simulink model "main"  (Simulink 8.1)
settings: Solver=ode4  StartTime=0  StopTime=0.2  FixedStep=Ts  MaxStep=1e-6  RelTol=1e-6  AbsTol=1e-6
PreLoadFcn:
  | assignin('base','Ts',[5e-6])
  | Ki=16.61;
  | Kp=0.013;
undefined symbols (not defined in the file): Ts
libraries: simulink x12, powerlib x11
Description:
  | This demonstration illustrates use of the BLDC in a closed-loop
  | speed and voltage control on a 1 kW, 3000 rpm industrial motor
  | 
  | 
  | Copyright 2008-2009 The MathWorks(TM), Inc.
settings Model: Creator=Olivier Tremblay  LastModifiedBy=The  ExtModeAutoUpdateStatusClock=off
settings DataIOCC: SignalLoggingName=sigsOut
settings OptimizationCC: InitFltsAndDblsToZero=on
settings DebuggingCC: SignalResolutionControl=TryResolveAllWithWarning  SolverPrmCheckMsg=none  MultiTaskDSMMsg=warning  MultiTaskCondExecSysMsg=none  UnknownTsInhSupMsg=none  StrictBusMsg=None
settings HardwareCC: TargetUnknown=on
settings RTWCC: IncludeERTFirstTime=on

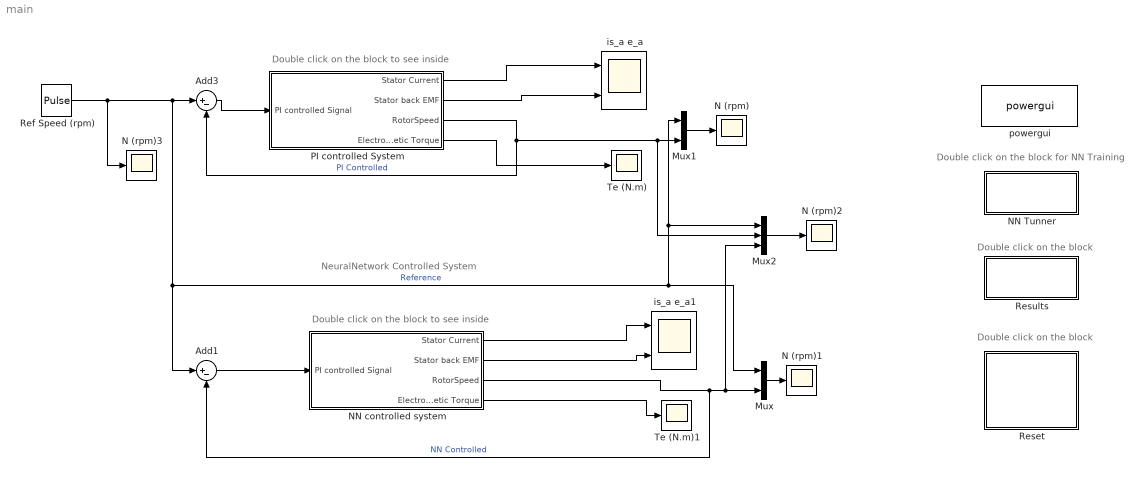
== system main ==
  note: Double click on the block for NN Training
  note: NeuralNetwork Controlled System
  note: Double click on the block to see inside
  note: Double click on the block to see inside
  note: Double click on the block
  note: Double click on the block
  Add1 : Sum  Inputs=|+-
  Add3 : Sum  Inputs=|+-
  Mux : Mux  Inputs=2
  Mux1 : Mux  Inputs=2
  Mux2 : Mux  Inputs=3
  N (rpm){,1..3} (4 alike) : Scope
      N (rpm) settings: TimeRange=0.2  YMin=0  YMax=3500  SaveName=N
      N (rpm)1 settings: TimeRange=0.2  YMin=0  YMax=3500  SaveName=N2
      N (rpm)2 settings: TimeRange=0.2  YMin=0  YMax=3500  SaveName=N4
      N (rpm)3 settings: TimeRange=0.2  YMin=0  YMax=3500  SaveName=N5
  NN Tunner : Subsystem
      settings: OpenFcn=|
      | Ki=16.61;Kp=.013;
      | Ts=5e-6;
      | options=simset('solver','ode45','srcWorkspace','Current','DstWorkspace','Current');
      | sim('Refmodel.slx',[0,0.1],options);
      | a=N.signals.values(:,1);
      | b=in.*ones(numel(a),1);
      | net = newff(minmax(a'),[2,1],{'tansig','purelin'},'trainlm');
      | net.trainParam.epochs=10;
      | net.trainParam.lr = 0.3;
      | [net,tr]=train(net,a',b');
      | x=sim(net,a');
      | Ki=abs(net.b{1,1}(1));
      | Kp=abs(net.b{1,1}(2));
      mask Display: image('nn.jpg')
  NN controlled system : Subsystem
  PI controlled System : Subsystem
  Ref Speed (rpm) : DiscretePulseGenerator  PulseType=Time based  Amplitude=3000  Period=0.1  PulseWidth=5
  Reset : Subsystem
      settings: OpenFcn=|
      | clear all
      | close all
      | Ki=16.61;Kp=.013;
      | Ts=5e-6;
      mask Display: image('reset.jpg')
  Results : Subsystem
      settings: OpenFcn=|
      | figure
      | plot(N.time,N.signals.values(:,1),N.time,N.signals.values(:,2),'r','LineWidth',2)
      | hold on
      | plot(N2.time,N2.signals.values(:,2),'g','LineWidth',2)
      | legend('Reference Speed','PI controlled Speed','NN Controlled Speed','Position','SouthEast')
      | xlabel('Time in secs')
      | ylabel('Speed in rpm')
      | title('Speed vs Time Curve')
      | grid on
      | 
      | 
      | figure
      | plot(N1.time,N1.signals.values,N3.time,N3.signals.values,'r','LineWidth',2)
      | xlabel('Times in sec')
      | ylabel('Torque in N.m')
      | legend('PI Controlled','NN Controlled','Position')
      | grid on
      | title('Torque vs Time curve')
      mask Display: image('results.jpg')
  Te (N.m) : Scope
      settings: TimeRange=0.2  YMin=0  YMax=3500  SaveName=N1
  Te (N.m)1 : Scope
      settings: TimeRange=0.2  YMin=0  YMax=3500  SaveName=N3
  is_a e_a : Scope  NumInputPorts=2
      settings: TimeRange=0.2  YMin=-15~-250  YMax=20~250  SaveName=IE
  is_a e_a1 : Scope  NumInputPorts=2
      settings: TimeRange=0.2  YMin=-15~-250  YMax=20~250  SaveName=IE1
  powergui : powerlib/powergui  Priority=2  SimulationMode=Discrete  SolverType=Tustin  SampleTime=Ts  frequency=60  SPID=off  DisableSnubberDevices=off  DisableRonSwitches=off  DisableVfSwitches=off  SwTol=0  Interpol=off  DisplayEquations=off  frequencyindice=0  Pbase=100e6  ErrMax=1e-4  Iterations=50  UnitsV=kV  UnitsW=MW  FunctionMessages=off  echomessages=off  HookPort=off  EnableUseOfTLC=off  x0status=blocks  RestoreLinks=warning  ResistiveCurrentMeasurement=off  Frange=[0:2:500]  Ylog=off  Xlog=on  ShowGrid=off  save=off  variable=ZData  ZoomFFT=on  StartTime=0.0  cycles=1  DisplayStyle=1  fundamental=60  FreqAxis=off  MaxFrequency=1000  frequencyindicesteady=1  RmsSteady=1  display=off  Ts=0  methode=off
  wires:
  PI controlled System/1(Stator Current) -> is_a e_a/1
  PI controlled System/2(Stator back EMF) -> is_a e_a/2
  PI controlled System/3(RotorSpeed) -> Mux2/2, Mux1/2, Add3/2  "PI Controlled"
  PI controlled System/4(Electromagnetic Torque) -> Te (N.m)/1
  Add1/1 -> NN controlled system/1(PI controlled Signal)
  Add3/1 -> PI controlled System/1(PI controlled Signal)
  NN controlled system/1(Stator Current) -> is_a e_a1/1
  NN controlled system/4(Electromagnetic Torque) -> Te (N.m)1/1
  NN controlled system/2(Stator back EMF) -> is_a e_a1/2
  Ref Speed (rpm)/1 -> N (rpm)3/1, Add1/1, Mux2/1, Mux1/1, Mux/1, Add3/1  "Reference"
  Mux/1 -> N (rpm)1/1
  NN controlled system/3(RotorSpeed) -> Mux2/3, Mux/2, Add1/2  "NN Controlled"
  Mux1/1 -> N (rpm)/1
  Mux2/1 -> N (rpm)2/1

== system main/NN Tunner ==

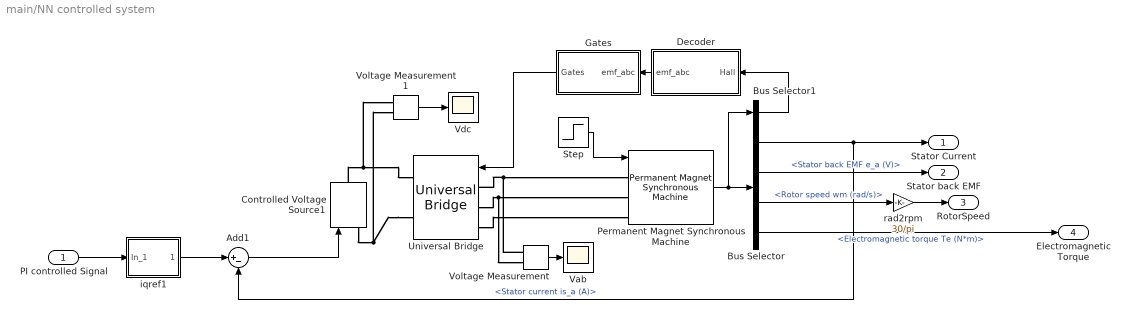
== system main/NN controlled system ==
  PI controlled Signal : Inport
  Add1 : Sum  Inputs=|+-
  Bus Selector : BusSelector  OutputSignals=Stator current is_a (A),Stator back EMF e_a (V),Rotor speed wm (rad/s),Electromagnetic torque Te (N*m)
  Bus Selector1 : BusSelector  OutputSignals=Hall effect signal h_a,Hall effect signal h_b,Hall effect signal h_c  OutputAsBus=on
  Controlled Voltage Source1 : powerlib/Electrical Sources/Controlled Voltage Source  Initialize=on  Source_Type=AC  Amplitude=500  Phase=0  Frequency=0  Measurements=None
  Decoder : Subsystem
  Gates : Subsystem
  Permanent Magnet Synchronous Machine : powerlib/Machines/Permanent Magnet Synchronous Machine  NbPhases=3  FluxDistribution=Trapezoidal  RotorType=Round  MechanicalLoad=Torque Tm  PresetModel=No  ShowDetailedParameters=on  Resistance=2.8750  Inductance=8.5e-3  dqInductances=[8.5e-3, 8.5e-3]  La=0.000835  MachineConstant=Flux linkage established by magnets (V.s)  Flux=0.175  VoltageCst=146.6077  TorqueCst=1.4  Flat=120  Mechanical="[ 0.8e-3, 1e-3,  4 ]"  PolePairs=4  InitialConditions=[0,0, 0,0]  InitialConditions5ph=[0 0 0 0 0 0]  TsPowergui=0  TsBlock=-1  RefAngle=90 degrees behind phase A axis (modified Park)
  Step : Step  Time=.1  After=3  SampleTime=Ts
  Universal Bridge : powerlib/Power Electronics/Universal Bridge  Arms=3  SnubberResistance=5000  SnubberCapacitance=1e-6  Device=MOSFET / Diodes  Ron=1e-3  Lon=0  ForwardVoltages="[  0  0  ]"  ForwardVoltage=0  GTOparameters=[ 10e-6 , 20e-6 ]  IGBTparameters=[ 1e-6 , 2e-6 ]  Measurements=None  Measurements_2=None  converterType=Rectifier
  Vab : Scope
      settings: TimeRange=0.06  YMin=-10000  YMax=10000  DataFormat=Structure
  Vdc : Scope
      settings: TimeRange=0.2  YMin=0  YMax=500  DataFormat=Structure
  Voltage Measurement : powerlib/Measurements/Voltage Measurement  PhasorSimulation=off  OutputType=Complex  PSBequivalent=0
  Voltage Measurement1 : powerlib/Measurements/Voltage Measurement  PhasorSimulation=off  OutputType=Complex  PSBequivalent=0
  iqref1 : Subsystem  mask(PI Controller){I=Ki, P=Kp, sat=[-500, 500]}
      mask prompts: I "Integral"; P "Proportional:"; sat "Minimum and maximum outputs:"
      mask init:
      | min=sat(1);max=sat(2);
      mask Display: disp('PI')
  rad2rpm : Gain  Gain=30/pi
  Stator Current : Outport
  Stator back EMF : Outport  Port=2
  RotorSpeed : Outport  Port=3
  Electromagnetic Torque : Outport  Port=4
  wires:
  Step/1 -> Permanent Magnet Synchronous Machine/1
  Gates/1(Gates) -> Universal Bridge/1
  Decoder/1(emf_abc) -> Gates/1("emf_abc ")
  Voltage Measurement/1 -> Vab/1
  Voltage Measurement1/1 -> Vdc/1
  Bus Selector/1 -> Add1/2, Stator Current/1  "<Stator current is_a (A)>"
  Permanent Magnet Synchronous Machine/1 -> Bus Selector/1, Bus Selector1/1
  Bus Selector1/1 -> Decoder/1("Hall ")
  Bus Selector/2 -> Stator back EMF/1  "<Stator back EMF e_a (V)>"
  Bus Selector/3 -> rad2rpm/1  "<Rotor speed wm (rad/s)>"
  Bus Selector/4 -> Electromagnetic Torque/1  "<Electromagnetic torque Te (N*m)>"
  rad2rpm/1 -> RotorSpeed/1
  PI controlled Signal/1 -> iqref1/1(In_1)
  Add1/1 -> Controlled Voltage Source1/1
  iqref1/1(Out_1) -> Add1/1
  connections:
  Voltage Measurement/LConn1 -- Universal Bridge/LConn1 -- Permanent Magnet Synchronous Machine/LConn1
  Universal Bridge/LConn2 -- Voltage Measurement/LConn2 -- Permanent Magnet Synchronous Machine/LConn2
  Universal Bridge/RConn1 -- Voltage Measurement1/LConn1 -- Controlled Voltage Source1/RConn1
  Universal Bridge/RConn2 -- Voltage Measurement1/LConn2 -- Controlled Voltage Source1/LConn1
  Universal Bridge/LConn3 -- Permanent Magnet Synchronous Machine/LConn3

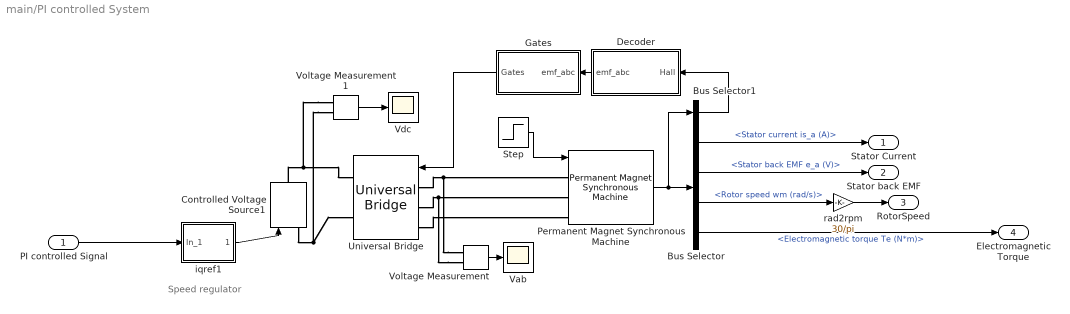
== system main/PI controlled System ==
  note: Speed
      | regulator
  PI controlled Signal : Inport
  Bus Selector : BusSelector  OutputSignals=Stator current is_a (A),Stator back EMF e_a (V),Rotor speed wm (rad/s),Electromagnetic torque Te (N*m)
  Bus Selector1 : BusSelector  OutputSignals=Hall effect signal h_a,Hall effect signal h_b,Hall effect signal h_c  OutputAsBus=on
  Controlled Voltage Source1 : powerlib/Electrical Sources/Controlled Voltage Source  Initialize=on  Source_Type=AC  Amplitude=500  Phase=0  Frequency=0  Measurements=None
  Decoder : Subsystem
  Gates : Subsystem
  Permanent Magnet Synchronous Machine : powerlib/Machines/Permanent Magnet Synchronous Machine  NbPhases=3  FluxDistribution=Trapezoidal  RotorType=Round  MechanicalLoad=Torque Tm  PresetModel=No  ShowDetailedParameters=on  Resistance=2.8750  Inductance=8.5e-3  dqInductances=[8.5e-3, 8.5e-3]  La=0.000835  MachineConstant=Flux linkage established by magnets (V.s)  Flux=0.175  VoltageCst=146.6077  TorqueCst=1.4  Flat=120  Mechanical="[ 0.8e-3, 1e-3,  4 ]"  PolePairs=4  InitialConditions=[0,0, 0,0]  InitialConditions5ph=[0 0 0 0 0 0]  TsPowergui=0  TsBlock=-1  RefAngle=90 degrees behind phase A axis (modified Park)
  Step : Step  Time=.1  After=3  SampleTime=0
  Universal Bridge : powerlib/Power Electronics/Universal Bridge  Arms=3  SnubberResistance=5000  SnubberCapacitance=1e-6  Device=MOSFET / Diodes  Ron=1e-3  Lon=0  ForwardVoltages="[  0  0  ]"  ForwardVoltage=0  GTOparameters=[ 10e-6 , 20e-6 ]  IGBTparameters=[ 1e-6 , 2e-6 ]  Measurements=None  Measurements_2=None  converterType=Rectifier
  Vab : Scope
      settings: TimeRange=0.06  YMin=-10000  YMax=10000  DataFormat=Structure
  Vdc : Scope
      settings: TimeRange=0.2  YMin=0  YMax=500  DataFormat=Structure
  Voltage Measurement : powerlib/Measurements/Voltage Measurement  PhasorSimulation=off  OutputType=Complex  PSBequivalent=0
  Voltage Measurement1 : powerlib/Measurements/Voltage Measurement  PhasorSimulation=off  OutputType=Complex  PSBequivalent=0
  iqref1 : Subsystem  mask(PI Controller){I=16.61, P=.013, sat=[-500, 500]}
      mask prompts: I "Integral"; P "Proportional:"; sat "Minimum and maximum outputs:"
      mask init:
      | min=sat(1);max=sat(2);
      mask Display: disp('PI')
  rad2rpm : Gain  Gain=30/pi
  Stator Current : Outport
  Stator back EMF : Outport  Port=2
  RotorSpeed : Outport  Port=3
  Electromagnetic Torque : Outport  Port=4
  wires:
  Step/1 -> Permanent Magnet Synchronous Machine/1
  iqref1/1(Out_1) -> Controlled Voltage Source1/1
  Gates/1(Gates) -> Universal Bridge/1
  Decoder/1(emf_abc) -> Gates/1("emf_abc ")
  Voltage Measurement/1 -> Vab/1
  Voltage Measurement1/1 -> Vdc/1
  Bus Selector/1 -> Stator Current/1  "<Stator current is_a (A)>"
  Permanent Magnet Synchronous Machine/1 -> Bus Selector/1, Bus Selector1/1
  Bus Selector1/1 -> Decoder/1("Hall ")
  Bus Selector/2 -> Stator back EMF/1  "<Stator back EMF e_a (V)>"
  Bus Selector/3 -> rad2rpm/1  "<Rotor speed wm (rad/s)>"
  Bus Selector/4 -> Electromagnetic Torque/1  "<Electromagnetic torque Te (N*m)>"
  rad2rpm/1 -> RotorSpeed/1
  PI controlled Signal/1 -> iqref1/1(In_1)
  connections:
  Voltage Measurement/LConn1 -- Permanent Magnet Synchronous Machine/LConn1 -- Universal Bridge/LConn1
  Voltage Measurement/LConn2 -- Permanent Magnet Synchronous Machine/LConn2 -- Universal Bridge/LConn2
  Voltage Measurement1/LConn1 -- Controlled Voltage Source1/RConn1 -- Universal Bridge/RConn1
  Voltage Measurement1/LConn2 -- Controlled Voltage Source1/LConn1 -- Universal Bridge/RConn2
  Universal Bridge/LConn3 -- Permanent Magnet Synchronous Machine/LConn3

== system main/Reset ==

== system main/Results ==

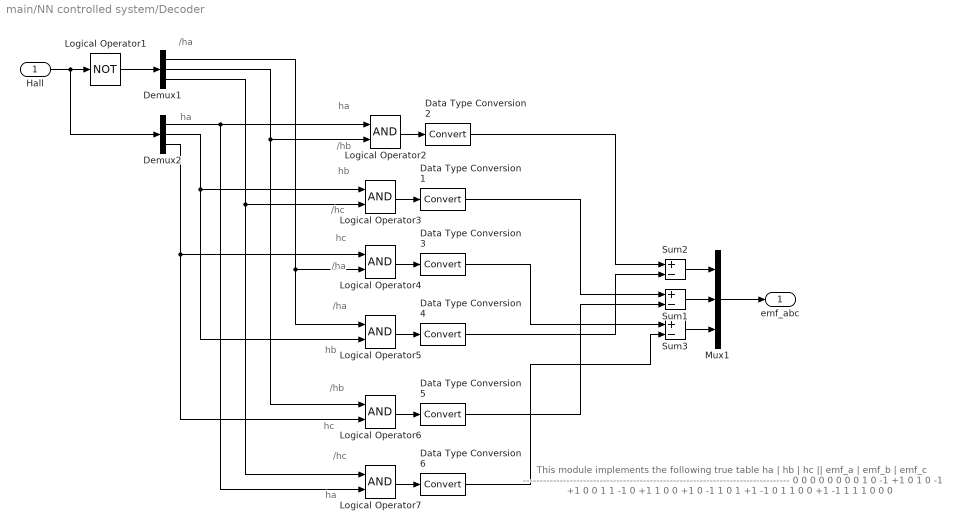
== system main/NN controlled system/Decoder ==
  note: /ha
  note: ha
  note: ha
  note: /hb
  note: hb
  note: /hc
  note: hc
  note: /ha
  note: /ha
  note: hb
  note: /hb
  note: hc
  note: /hc
  note: ha
  note: This module implements the following true table
      |
      |    ha   |   hb   |   hc   ||   emf_a   |   emf_b   |   emf_c
      |     --------------------------------------------------------------------------------
      | 0          0         0          0               0               0
      | 0          0         1          0               -1              +1
      | 0          1         0          -1              +1                0
      | 0          1         1          -1               0               +1
      | 1          0         0         +1               0               -1
      | 1          0         1         +1              -1                0
      | 1          1         0          0              +1               -1
      | 1          1         1          0               0                0
  "Hall " : Inport
  Data Type Conversion{1..6} (6 alike) : DataTypeConversion
  Demux1 : Demux  Outputs=3
  Demux2 : Demux  Outputs=3
  Logical Operator1 : Logic  Operator=NOT  AllPortsSameDT=off  OutDataTypeStr=boolean
  Logical Operator{2..7} (6 alike) : Logic  AllPortsSameDT=off  OutDataTypeStr=boolean
  Mux1 : Mux  Inputs=3
  Sum1 : Sum  Inputs=+-  OutDataTypeStr=double
  Sum2 : Sum  Inputs=+-  OutDataTypeStr=double
  Sum3 : Sum  Inputs=+-  OutDataTypeStr=double
  emf_abc : Outport
  wires:
  "Hall "/1 -> Logical Operator1/1, Demux2/1
  Logical Operator1/1 -> Demux1/1
  Demux2/3 -> Logical Operator4/1, Logical Operator6/2
  Demux2/2 -> Logical Operator3/1, Logical Operator5/2
  Demux2/1 -> Logical Operator2/1, Logical Operator7/2
  Demux1/3 -> Logical Operator3/2, Logical Operator7/1
  Demux1/2 -> Logical Operator2/2, Logical Operator6/1
  Demux1/1 -> Logical Operator4/2, Logical Operator5/1
  Logical Operator2/1 -> Data Type Conversion2/1
  Sum2/1 -> Mux1/1
  Sum1/1 -> Mux1/2
  Sum3/1 -> Mux1/3
  Mux1/1 -> emf_abc/1
  Logical Operator3/1 -> Data Type Conversion1/1
  Logical Operator4/1 -> Data Type Conversion3/1
  Logical Operator5/1 -> Data Type Conversion4/1
  Logical Operator6/1 -> Data Type Conversion5/1
  Logical Operator7/1 -> Data Type Conversion6/1
  Data Type Conversion2/1 -> Sum2/1
  Data Type Conversion4/1 -> Sum2/2
  Data Type Conversion1/1 -> Sum1/1
  Data Type Conversion5/1 -> Sum1/2
  Data Type Conversion3/1 -> Sum3/1
  Data Type Conversion6/1 -> Sum3/2

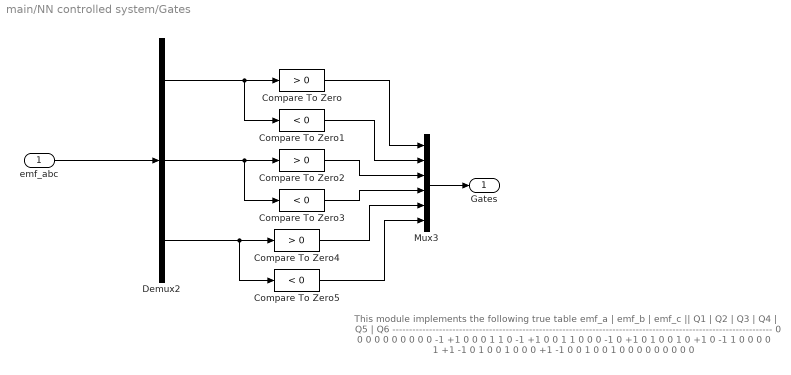
== system main/NN controlled system/Gates ==
  note: This module implements the following true table
      |
      |    emf_a   |   emf_b   |   emf_c   ||   Q1   |   Q2   |   Q3   |   Q4   |   Q5   |   Q6
      |     ------------------------------------------------------------------------------------------------------------------
      |       0              0                0            0          0          0           0        0        0
      |       0               -1              +1          0          0          0           1        1        0
      |     -1              +1                0          0          1          1           0        0        0
      |     -1               0               +1          0          1         0           0        1        0
      |    +1               0                -1          1          0          0           0        0        1
      |    +1              -1                0           1          0          0           1        0        0
      |      0              +1               -1           0          0          1           0        0        1
      |     0              0                0             0          0          0           0        0        0
  "emf_abc " : Inport
  Compare To Zero : simulink/Logic and Bit Operations/Compare To Zero  relop=>  OutDataTypeStr=boolean  ZeroCross=off
  Compare To Zero1 : simulink/Logic and Bit Operations/Compare To Zero  relop=<  OutDataTypeStr=boolean  ZeroCross=off
  Compare To Zero2 : simulink/Logic and Bit Operations/Compare To Zero  relop=>  OutDataTypeStr=boolean  ZeroCross=off
  Compare To Zero3 : simulink/Logic and Bit Operations/Compare To Zero  relop=<  OutDataTypeStr=boolean  ZeroCross=off
  Compare To Zero4 : simulink/Logic and Bit Operations/Compare To Zero  relop=>  OutDataTypeStr=boolean  ZeroCross=off
  Compare To Zero5 : simulink/Logic and Bit Operations/Compare To Zero  relop=<  OutDataTypeStr=boolean  ZeroCross=off
  Demux2 : Demux  Outputs=3
  Mux3 : Mux  Inputs=6
  Gates : Outport
  wires:
  "emf_abc "/1 -> Demux2/1
  Mux3/1 -> Gates/1
  Demux2/1 -> Compare To Zero/1, Compare To Zero1/1
  Demux2/2 -> Compare To Zero2/1, Compare To Zero3/1
  Demux2/3 -> Compare To Zero4/1, Compare To Zero5/1
  Compare To Zero/1 -> Mux3/1
  Compare To Zero1/1 -> Mux3/2
  Compare To Zero2/1 -> Mux3/3
  Compare To Zero3/1 -> Mux3/4
  Compare To Zero4/1 -> Mux3/5
  Compare To Zero5/1 -> Mux3/6

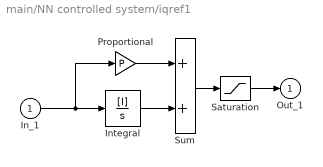
== system main/NN controlled system/iqref1 ==
  In_1 : Inport
  Integral : TransferFcn  Numerator=[I]  Denominator=[1 0]
  Proportional : Gain  Gain=P  SaturateOnIntegerOverflow=on  OutDataTypeStr=Inherit: Same as input  ParamDataTypeStr=Inherit: Same as input
  Saturation : Saturate  UpperLimit=max  LowerLimit=min
  Sum : Sum  SaturateOnIntegerOverflow=on  InputSameDT=on  OutDataTypeStr=Inherit: Same as first input
  Out_1 : Outport  InitialOutput=0
  wires:
  Saturation/1 -> Out_1/1
  Sum/1 -> Saturation/1
  Proportional/1 -> Sum/1
  In_1/1 -> Proportional/1, Integral/1
  Integral/1 -> Sum/2

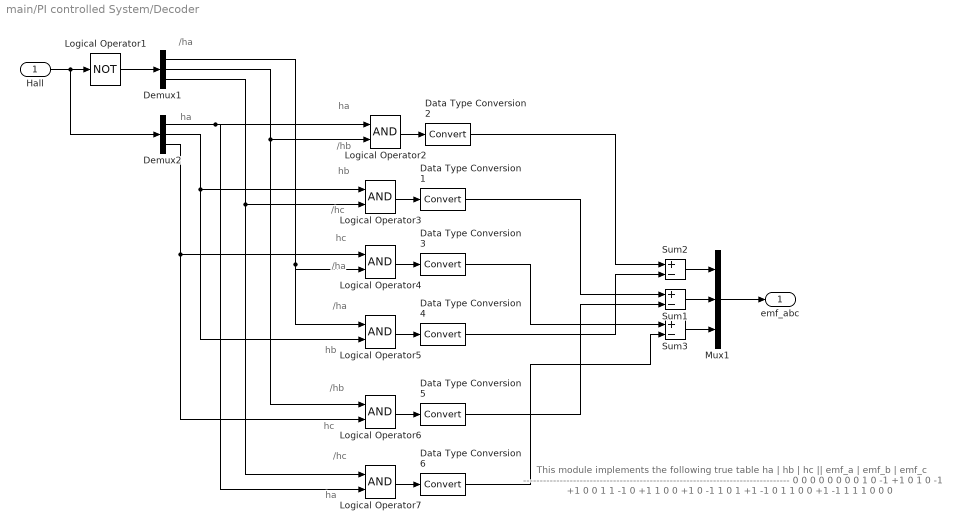
== system main/PI controlled System/Decoder ==
  note: /ha
  note: ha
  note: ha
  note: /hb
  note: hb
  note: /hc
  note: hc
  note: /ha
  note: /ha
  note: hb
  note: /hb
  note: hc
  note: /hc
  note: ha
  note: This module implements the following true table
      |
      |    ha   |   hb   |   hc   ||   emf_a   |   emf_b   |   emf_c
      |     --------------------------------------------------------------------------------
      | 0          0         0          0               0               0
      | 0          0         1          0               -1              +1
      | 0          1         0          -1              +1                0
      | 0          1         1          -1               0               +1
      | 1          0         0         +1               0               -1
      | 1          0         1         +1              -1                0
      | 1          1         0          0              +1               -1
      | 1          1         1          0               0                0
  "Hall " : Inport
  Data Type Conversion{1..6} (6 alike) : DataTypeConversion
  Demux1 : Demux  Outputs=3
  Demux2 : Demux  Outputs=3
  Logical Operator1 : Logic  Operator=NOT  AllPortsSameDT=off  OutDataTypeStr=boolean
  Logical Operator{2..7} (6 alike) : Logic  AllPortsSameDT=off  OutDataTypeStr=boolean
  Mux1 : Mux  Inputs=3
  Sum1 : Sum  Inputs=+-  OutDataTypeStr=double
  Sum2 : Sum  Inputs=+-  OutDataTypeStr=double
  Sum3 : Sum  Inputs=+-  OutDataTypeStr=double
  emf_abc : Outport
  wires:
  "Hall "/1 -> Logical Operator1/1, Demux2/1
  Logical Operator1/1 -> Demux1/1
  Demux2/3 -> Logical Operator4/1, Logical Operator6/2
  Demux2/2 -> Logical Operator3/1, Logical Operator5/2
  Demux2/1 -> Logical Operator2/1, Logical Operator7/2
  Demux1/3 -> Logical Operator3/2, Logical Operator7/1
  Demux1/2 -> Logical Operator2/2, Logical Operator6/1
  Demux1/1 -> Logical Operator4/2, Logical Operator5/1
  Logical Operator2/1 -> Data Type Conversion2/1
  Sum2/1 -> Mux1/1
  Sum1/1 -> Mux1/2
  Sum3/1 -> Mux1/3
  Mux1/1 -> emf_abc/1
  Logical Operator3/1 -> Data Type Conversion1/1
  Logical Operator4/1 -> Data Type Conversion3/1
  Logical Operator5/1 -> Data Type Conversion4/1
  Logical Operator6/1 -> Data Type Conversion5/1
  Logical Operator7/1 -> Data Type Conversion6/1
  Data Type Conversion2/1 -> Sum2/1
  Data Type Conversion4/1 -> Sum2/2
  Data Type Conversion1/1 -> Sum1/1
  Data Type Conversion5/1 -> Sum1/2
  Data Type Conversion3/1 -> Sum3/1
  Data Type Conversion6/1 -> Sum3/2

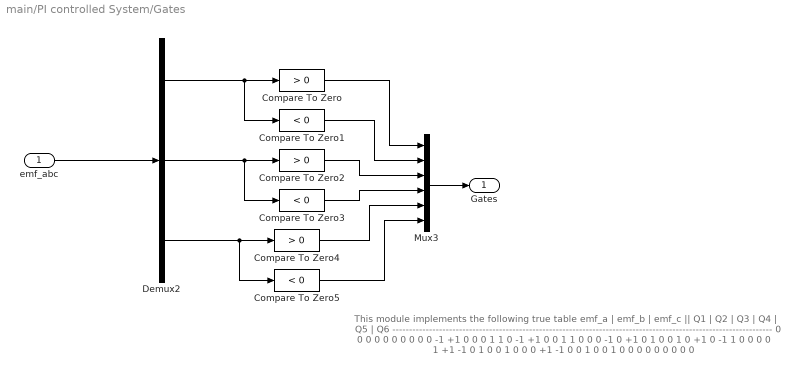
== system main/PI controlled System/Gates ==
  note: This module implements the following true table
      |
      |    emf_a   |   emf_b   |   emf_c   ||   Q1   |   Q2   |   Q3   |   Q4   |   Q5   |   Q6
      |     ------------------------------------------------------------------------------------------------------------------
      |       0              0                0            0          0          0           0        0        0
      |       0               -1              +1          0          0          0           1        1        0
      |     -1              +1                0          0          1          1           0        0        0
      |     -1               0               +1          0          1         0           0        1        0
      |    +1               0                -1          1          0          0           0        0        1
      |    +1              -1                0           1          0          0           1        0        0
      |      0              +1               -1           0          0          1           0        0        1
      |     0              0                0             0          0          0           0        0        0
  "emf_abc " : Inport
  Compare To Zero : simulink/Logic and Bit Operations/Compare To Zero  relop=>  OutDataTypeStr=boolean  ZeroCross=off
  Compare To Zero1 : simulink/Logic and Bit Operations/Compare To Zero  relop=<  OutDataTypeStr=boolean  ZeroCross=off
  Compare To Zero2 : simulink/Logic and Bit Operations/Compare To Zero  relop=>  OutDataTypeStr=boolean  ZeroCross=off
  Compare To Zero3 : simulink/Logic and Bit Operations/Compare To Zero  relop=<  OutDataTypeStr=boolean  ZeroCross=off
  Compare To Zero4 : simulink/Logic and Bit Operations/Compare To Zero  relop=>  OutDataTypeStr=boolean  ZeroCross=off
  Compare To Zero5 : simulink/Logic and Bit Operations/Compare To Zero  relop=<  OutDataTypeStr=boolean  ZeroCross=off
  Demux2 : Demux  Outputs=3
  Mux3 : Mux  Inputs=6
  Gates : Outport
  wires:
  "emf_abc "/1 -> Demux2/1
  Mux3/1 -> Gates/1
  Demux2/1 -> Compare To Zero/1, Compare To Zero1/1
  Demux2/2 -> Compare To Zero2/1, Compare To Zero3/1
  Demux2/3 -> Compare To Zero4/1, Compare To Zero5/1
  Compare To Zero/1 -> Mux3/1
  Compare To Zero1/1 -> Mux3/2
  Compare To Zero2/1 -> Mux3/3
  Compare To Zero3/1 -> Mux3/4
  Compare To Zero4/1 -> Mux3/5
  Compare To Zero5/1 -> Mux3/6

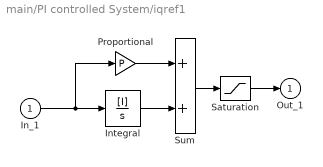
== system main/PI controlled System/iqref1 ==
  In_1 : Inport
  Integral : TransferFcn  Numerator=[I]  Denominator=[1 0]
  Proportional : Gain  Gain=P  SaturateOnIntegerOverflow=on  OutDataTypeStr=Inherit: Same as input  ParamDataTypeStr=Inherit: Same as input
  Saturation : Saturate  UpperLimit=max  LowerLimit=min
  Sum : Sum  SaturateOnIntegerOverflow=on  InputSameDT=on  OutDataTypeStr=Inherit: Same as first input
  Out_1 : Outport  InitialOutput=0
  wires:
  Saturation/1 -> Out_1/1
  Sum/1 -> Saturation/1
  Proportional/1 -> Sum/1
  In_1/1 -> Proportional/1, Integral/1
  Integral/1 -> Sum/2
